simulink model "dcmtrCtrl_PID_Harness1"  (R2025b)
settings: Solver=ode15s  StartTime=0.0  StopTime=13  RelTol=1e-3
libraries: simulink_extras x1, SignalEditorBlockLib x1
settings Model: DataDictionary=dcmtr_ctrl.sldd  Creator=smuckati  LastModifiedBy=jkhoury
settings OptimizationCC: DefaultParameterBehavior=Inlined  UseDivisionForNetSlopeComputation=on  EnhancedBackFolding=on  PassReuseOutputArgsAs=Individual arguments  ZeroExternalMemoryAtStartup=off  ZeroInternalMemoryAtStartup=off  OptimizeBlockOrder=speed  DifferentSizesBufferReuse=on  OptimizationCustomize=off  EfficientTunableParamExpr=on
settings DebuggingCC: SignalRangeChecking=error  ParameterPrecisionLossMsg=none  ParameterTunabilityLossMsg=error  UnconnectedInputMsg=warning  UnconnectedOutputMsg=warning  UnconnectedLineMsg=warning
settings ModelReferenceCC: EnableRefExpFcnMdlSchedulingChecks=on
settings SFSimCC: MATLABDynamicMemAlloc=off
settings RTWCC: SystemTargetFile=ert.tlc  GenCodeOnly=on  TemplateMakefile=ert_default_tmf  CodeExecutionProfiling=on  CodeProfilingSaveOptions=AllData  CodeProfilingInstrumentation=detailed  GPUComputeCapability=3.5  DLArmComputeVersion=19.05  Description=Embedded Coder
settings CodeAppCC: ForceParamTrailComments=on  IgnoreCustomStorageClasses=off  OperatorAnnotations=on  SimulinkDataObjDesc=on  SFDataObjDesc=on  InsertBlockDesc=on
settings ERTTargetCC: ERTCustomFileTemplate=example_file_process.tlc  DynamicArrayContainerType=coder::array  TargetLangStandard=C99 (ISO)  GenerateSampleERTMain=on

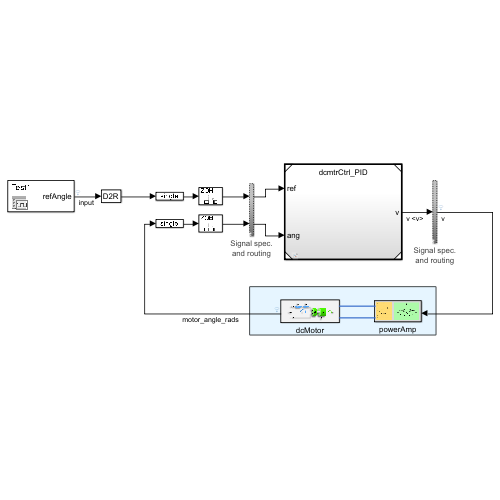
[thumbnail: Simulink's stored preview of the top-level diagram]
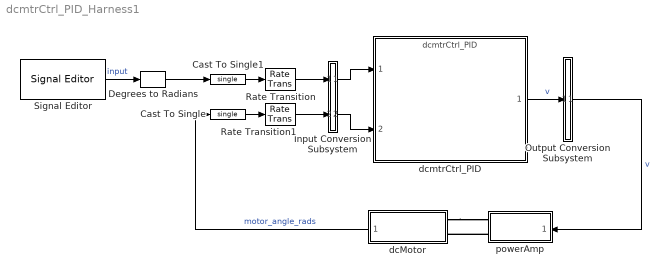
== system dcmtrCtrl_PID_Harness1 ==
  Cast To Single : DataTypeConversion  OutDataTypeStr=single  SaturateOnIntegerOverflow=off  RndMeth=Floor
  Cast To Single1 : DataTypeConversion  OutDataTypeStr=single  SaturateOnIntegerOverflow=off  RndMeth=Floor
  Degrees to Radians : simulink_extras/Transformations/Degrees to Radians
  Input Conversion Subsystem : Subsystem  Tag=__SLT_ICS__  Description=|
      | Signal spec.
      | and routing
      settings: AttributesFormatString=%<Description>
  Output Conversion Subsystem : Subsystem  Tag=__SLT_OCS__  Description=|
      | Signal spec.
      | and routing
      settings: AttributesFormatString=%<Description>
  Rate Transition : RateTransition  OutPortSampleTime=Ctrl_Ts
  Rate Transition1 : RateTransition  OutPortSampleTime=Ctrl_Ts
  Signal Editor : SignalEditorBlockLib/Signal Editor  FileName=dcmtrCtrl_testRefAngles.mat  ActiveScenario=Test1  ActiveSignal=refAngle  IsBus=off  OutputBusObjectStr=Bus: BusObject  SampleTime=0  ZeroCross=off  OutputAfterFinalValue=Setting to zero  Unit=inherit  PreserveSignalName=on  ApplySigPropsToAllScenarios=on  ApplySigPropsToAllSignals=off  SignalPropertySource=Dialog parameters
  dcMotor : Subsystem  ReferencedSubsystem=dcmtr
      settings: PermitHierarchicalResolution=None
  dcmtrCtrl_PID : ModelReference  ModelNameDialog=dcmtrCtrl_PID  SimulationMode=Normal  ModelReferenceVersion=9.4
  powerAmp : Subsystem  ReferencedSubsystem=powerAmp
  wires:
  Output Conversion Subsystem/1(Outport_1) -> powerAmp/1  "v"
  Input Conversion Subsystem/1(Outport_1) -> dcmtrCtrl_PID/1
  Input Conversion Subsystem/2(Outport_2) -> dcmtrCtrl_PID/2
  dcmtrCtrl_PID/1 -> Output Conversion Subsystem/1(Inport_1)  "v"
  Signal Editor/1 -> Degrees to Radians/1  "input"
  Cast To Single/1 -> Rate Transition1/1
  Cast To Single1/1 -> Rate Transition/1
  Degrees to Radians/1 -> Cast To Single1/1
  dcMotor/1 -> Cast To Single/1  "motor_angle_rads"
  Rate Transition/1 -> Input Conversion Subsystem/1(Inport_1)
  Rate Transition1/1 -> Input Conversion Subsystem/2(Inport_2)
  connections:
  dcMotor/LConn1 -- powerAmp/RConn1
  powerAmp/RConn2 -- dcMotor/LConn2

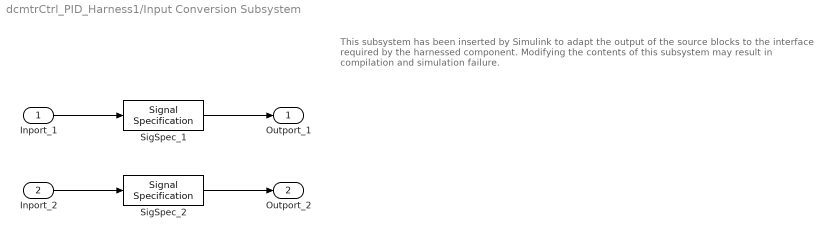
== system dcmtrCtrl_PID_Harness1/Input Conversion Subsystem ==
  note: This subsystem has been inserted by Simulink to adapt the output of the source blocks to the interface required by the harnessed component.
      |  Modifying the contents of this subsystem may result in compilation and simulation failure.
  Inport_1 : Inport
  Inport_2 : Inport  Port=2
  SigSpec_1 : SignalSpecification  OutDataTypeStr=single  Dimensions=[1]  SampleTime=0.01
  SigSpec_2 : SignalSpecification  OutDataTypeStr=single  Dimensions=[1]  SampleTime=0.01
  Outport_1 : Outport
  Outport_2 : Outport  Port=2
  wires:
  SigSpec_1/1 -> Outport_1/1
  Inport_1/1 -> SigSpec_1/1
  SigSpec_2/1 -> Outport_2/1
  Inport_2/1 -> SigSpec_2/1

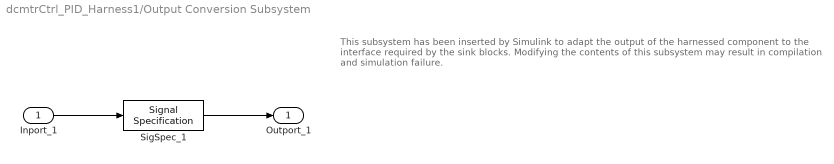
== system dcmtrCtrl_PID_Harness1/Output Conversion Subsystem ==
  note: This subsystem has been inserted by Simulink to adapt the output of the harnessed component to the interface required by the sink blocks.
      |  Modifying the contents of this subsystem may result in compilation and simulation failure.
  Inport_1 : Inport
  SigSpec_1 : SignalSpecification  OutDataTypeStr=single  Dimensions=[1]  SampleTime=0.01
  Outport_1 : Outport
  wires:
  Inport_1/1 -> SigSpec_1/1
  SigSpec_1/1 -> Outport_1/1
